simulink model "Rober"  (Simulink 10.0)
settings: Solver=ode45  StartTime=0.0  StopTime=40  RelTol=1e-3  EnableMultiTasking=on
settings Model: Creator=UX31  LastModifiedBy=unknown
settings DataIOCC: LimitDataPoints=on
settings DebuggingCC: UnderspecifiedInitializationDetection=Simplified  MergeDetectMultiDrivingBlocksExec=error  SolverPrmCheckMsg=warning
settings GRTTargetCC: GeneratePreprocessorConditionals=Disable all  CombineOutputUpdateFcns=on  GRTInterface=off
settings ConfigComp: CovExternalEMLEnable=off  CovSFcnEnable=off

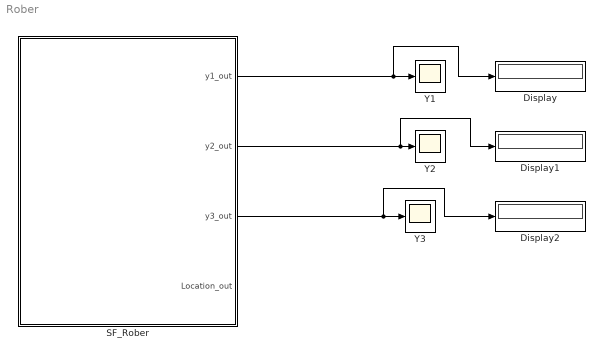
== system Rober ==
  Display : Display
  Display1 : Display
  Display2 : Display
  SF_Rober : Stateflow chart  TreatAsAtomicUnit=on
  Y1 : Scope
  Y2 : Scope
  Y3 : Scope
  wires:
  SF_Rober/3(y3_out) -> Display2/1, Y3/1
  SF_Rober/2(y2_out) -> Display1/1, Y2/1
  SF_Rober/1(y1_out) -> Display/1, Y1/1

== stateflow chart SF_Rober ==
  settings: updateMethod=CONTINUOUS
  state Rober
    du:
    y1_dot=(0-k1)*y1+k3*y2*y3;
    y2_dot=k1*y1-k2*y2*y2-k3*y2*y3;
    y3_dot=k2*y2^2;
    y1_out=y1;
    y2_out=y2;
    y3_out=y3;
    Location_out =1;
  (default) -> Rober : {y1= 1; y2 =0; y3 =0}
  data: y1 local double; y1_out output double; y2 local double; y2_out output double; y3 local double; y3_out output double; Location_out output double; k1 constant double =0.04; k2 constant double =3*10^7; k3 constant double =10^4
  data y1 settings: updateMethod=SF_CONTINUOUS_TIME_DATA
  data y2 settings: updateMethod=SF_CONTINUOUS_TIME_DATA
  data y3 settings: updateMethod=SF_CONTINUOUS_TIME_DATA
